simulink model "Final"  (R2021a)
settings: Solver=VariableStepAuto  StartTime=0.0  StopTime=1  RelTol=1e-3
undefined symbols (not defined in the file): Ion, Lithium
libraries: spsDiodeLib x7, spsSeriesRLCBranchLib x5, spsCurrentMeasurementLib x2, spsVoltageMeasurementLib x2, spsBatteryLib x1, spsMosfetLib x1, spsPVArrayLib x1, simulink x1, spsGroundLib x1, spsPermanentMagnetSynchronousMachineLib x1, spsThreePhaseVIMeasurementLib x1, spsWindTurbineLib x1
settings Model: Creator=Akashgowda  LastModifiedBy=Akashgowda

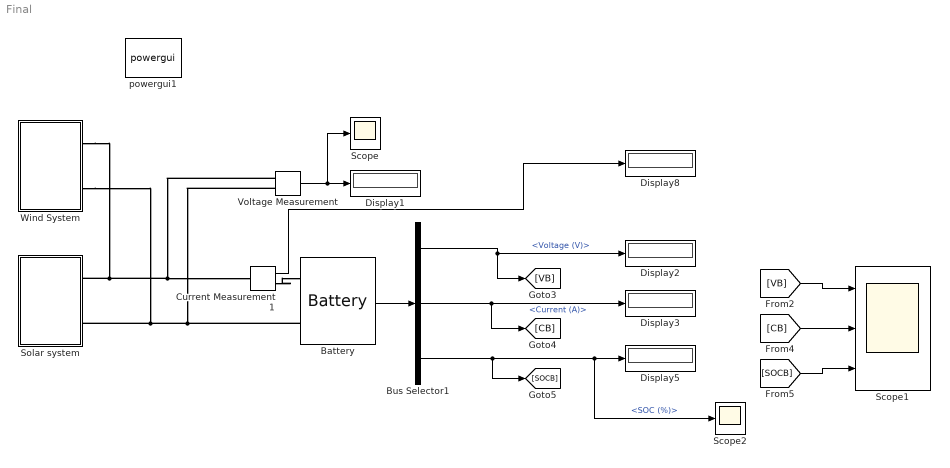
== system Final ==
  Battery : spsBatteryLib/Battery  BatType=Lithium-Ion  ShowTempParam=off  ThermalPreset=no  ShowAgeParam=off  NomV=12  NomQ=150  SOC=90  Batt_Tr=10  PresetModel=on  MaxQ=150  MinV=9  FullV=13.9678  Dis_rate=65.2174  R=0.0008  Normal_OP=135.6522  expZone="[12.9646      7.36957]"  current=[6.5 13 32.5]  Units=Time  Tci=20  NomT=20  T2=-30  MaxQ2=4.8  FullV2=7.1  Normal_OP2=5.655  expZone2="[6.58           1]"  Rca=0.6  ti=2000  Dp=0  Neq0=0  Tsim=1e6  Ta1=25  Qeol=5.4*0.9  Reol=0.013333*1.2  Char_age=[2.3478, 3]  Dis_age=[2.3478, 10]  N1=1500  N2=10500  N3=1000  N4=1400  Ta2=45  N5=950
  Bus Selector1 : BusSelector  OutputSignals=Voltage (V),Current (A),SOC (%)
  Current Measurement1 : spsCurrentMeasurementLib/Current Measurement  PhasorSimulation=off  OutputType=Complex  PSBequivalent=0
  Display{1..3,5,8} (5 alike) : Display
  Scope : Scope
  Scope1 : Scope  NumInputPorts=3
  Scope2 : Scope
  Solar system : Subsystem
  Voltage Measurement : spsVoltageMeasurementLib/Voltage Measurement  PhasorSimulation=off  OutputType=Complex  PSBequivalent=0
  Wind System : Subsystem
  powergui1 : spspowerguiLib/powergui  Priority=1  SimulationMode=Continuous  SampleTime=50e-6  frequency=60  Iterations=50  frequencyindice=0  Pbase=100e6  ErrMax=1e-4  UnitsV=kV  UnitsW=MW  buscounter=0  FunctionMessages=off  echomessages=off  EnableUseOfTLC=off  CurrentSourceSwitches=off  DisableSnubberDevices=off  DisableRonSwitches=off  DisableVfSwitches=off  DisplayEquations=off  AutomaticDiscreteSolvers=off  SolverType=Tustin/Backward Euler (TBE)  Interpol=off  ExternalGateDelay=off  methode=off  Ts=100  x0status=blocks  SPID=on  SwTol=0  HookPort=off  NonlinearTolerance=1e-4  nMaxIteration=100  ContinueOnMaxIteration=off  RestoreLinks=warning  ResistiveCurrentMeasurement=off  Frange=[0:2:500]  Ylog=off  Xlog=on  ShowGrid=off  save=off  variable=ZData  structure=0  ZoomFFT=off  StartTime=0.0  cycles=1  DisplayStyle=1  fundamental=60  FreqAxis=off  MaxFrequency=1000  frequencyindicesteady=1  RmsSteady=1  display=off
  wires:
  [VB] -> Scope1/1
  [SOCB] -> Scope1/3
  Bus Selector1/1 -> Display2/1, [VB]  "<Voltage (V)>"
  Bus Selector1/3 -> [SOCB], Scope2/1, Display5/1  "<SOC (%)>"
  Bus Selector1/2 -> [CB], Display3/1  "<Current (A)>"
  [CB] -> Scope1/2
  Battery/1 -> Bus Selector1/1
  Voltage Measurement/1 -> Scope/1, Display1/1
  Current Measurement1/1 -> Display8/1
  connections:
  Wind System/RConn2 -- Battery/LConn2 -- Voltage Measurement/LConn2 -- Solar system/RConn2
  Wind System/RConn1 -- Current Measurement1/LConn1 -- Voltage Measurement/LConn1 -- Solar system/RConn1
  Current Measurement1/RConn1 -- Battery/LConn1

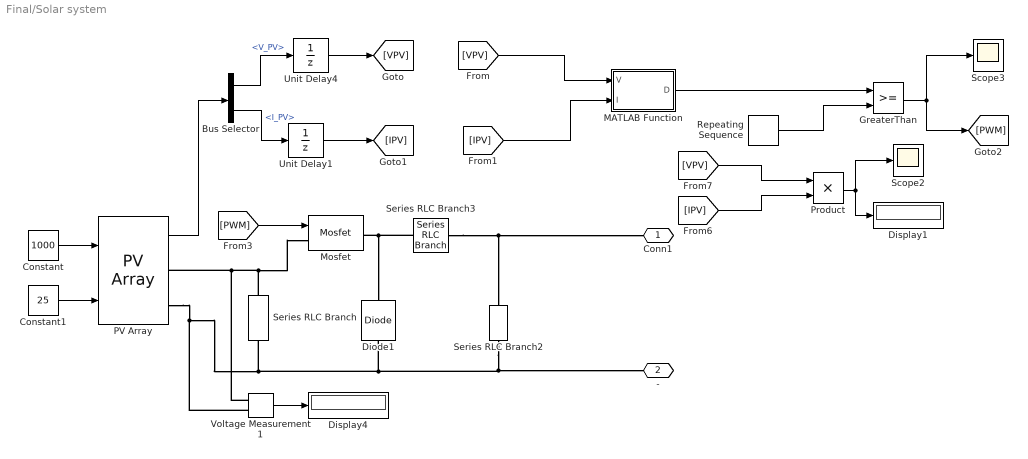
== system Final/Solar system ==
  Bus Selector : BusSelector  OutputSignals=V_PV,I_PV
  Constant : Constant  Value=1000
  Constant1 : Constant  Value=25
  Diode1 : spsDiodeLib/Diode  Ron=0.001  Lon=0  Vf=0.8  IC=0  UseSnubber=0  Rs=500  Cs=250e-9  Measurements=off
  Display1 : Display
  Display4 : Display
  GreaterThan : RelationalOperator  OutDataTypeStr=boolean  RndMeth=Simplest
  MATLAB Function : MATLAB Function  TreatAsAtomicUnit=on
  Mosfet : spsMosfetLib/Mosfet  Ron=0.1  Lon=0  Rd=0.01  Vfd=0  IC=0  Rs=1e5  Cs=inf  Measurements=off
  PV Array : spsPVArrayLib/PV Array  Npar=1  Nser=1  PlotType=array @ 25 deg.C & specified irradiances  S_vec="[ 1000  500  100 ]"  Temp_C_vec="[ 45 25  ]"  ModuleName=User-defined  PlotWhenSelected=off  Pm=213.15  Ncell=60  Voc=36.3  Isc=7.84  Vm=29  Im=7.35  beta_Voc_pc=-0.36099  alpha_Isc_pc=0.102  beta_Voc=-0.13104  alpha_Isc=0.0079968  IL=7.8654  I0=2.9273e-10  nI=0.98119  Rsh=313.0553  Rs=0.39381  RobustModel=off  RobustCellTemperature=313.3991  BAL=on  Tc=1e-6  Tfilter=5e-5
  Product : Product
  Repeating Sequence : simulink/Sources/Repeating Sequence  rep_seq_t=[0 0.0002]  rep_seq_y=[0 1]
  Scope2 : Scope
  Scope3 : Scope
  Series RLC Branch : spsSeriesRLCBranchLib/Series RLC Branch  LConnTagsString=__new0  RConnTagsString=__new0  BranchType=RC  Resistance=0.0001  Inductance=1e-3  SetiL0=off  InitialCurrent=0  Capacitance=1000e-6  Setx0=off  InitialVoltage=0  Measurements=None
  Series RLC Branch2 : spsSeriesRLCBranchLib/Series RLC Branch  LConnTagsString=__new0  RConnTagsString=__new0  BranchType=C  Resistance=1  Inductance=1e-3  SetiL0=off  InitialCurrent=0  Capacitance=369.79e-6  Setx0=off  InitialVoltage=0  Measurements=None
  Series RLC Branch3 : spsSeriesRLCBranchLib/Series RLC Branch  LConnTagsString=__new0  RConnTagsString=__new0  BranchType=L  Resistance=1  Inductance=772.64e-6  SetiL0=off  InitialCurrent=0  Capacitance=1e-6  Setx0=off  InitialVoltage=0  Measurements=None
  Unit Delay1 : UnitDelay  SampleTime=1e-4  HasFrameUpgradeWarning=on
  Unit Delay4 : UnitDelay  SampleTime=1e-4  HasFrameUpgradeWarning=on
  Voltage Measurement1 : spsVoltageMeasurementLib/Voltage Measurement  PhasorSimulation=off  OutputType=Complex  PSBequivalent=0
  Conn1 : PMIOPort  Side=Right
  - : PMIOPort  Port=2  Side=Right
  wires:
  Voltage Measurement1/1 -> Display4/1
  Constant/1 -> PV Array/1
  Bus Selector/2 -> Unit Delay1/1  "<I_PV>"
  Product/1 -> Display1/1, Scope2/1
  [IPV] -> Product/2
  PV Array/1 -> Bus Selector/1
  Constant1/1 -> PV Array/2
  Unit Delay4/1 -> [VPV]
  [VPV] -> Product/1
  Bus Selector/1 -> Unit Delay4/1  "<V_PV>"
  [VPV] -> MATLAB Function/1(V)
  Unit Delay1/1 -> [IPV]
  MATLAB Function/1(D) -> GreaterThan/1
  [IPV] -> MATLAB Function/2(I)
  Repeating Sequence/1 -> GreaterThan/2
  [PWM] -> Mosfet/1
  GreaterThan/1 -> Scope3/1, [PWM]
  connections:
  Series RLC Branch2/RConn1 -- PV Array/RConn2 -- Voltage Measurement1/LConn2 -- Series RLC Branch/RConn1 -- Diode1/LConn1 -- -/RConn1
  PV Array/RConn1 -- Series RLC Branch/LConn1 -- Mosfet/LConn1 -- Voltage Measurement1/LConn1
  Series RLC Branch3/RConn1 -- Mosfet/RConn1 -- Diode1/RConn1
  Series RLC Branch3/LConn1 -- Conn1/RConn1 -- Series RLC Branch2/LConn1

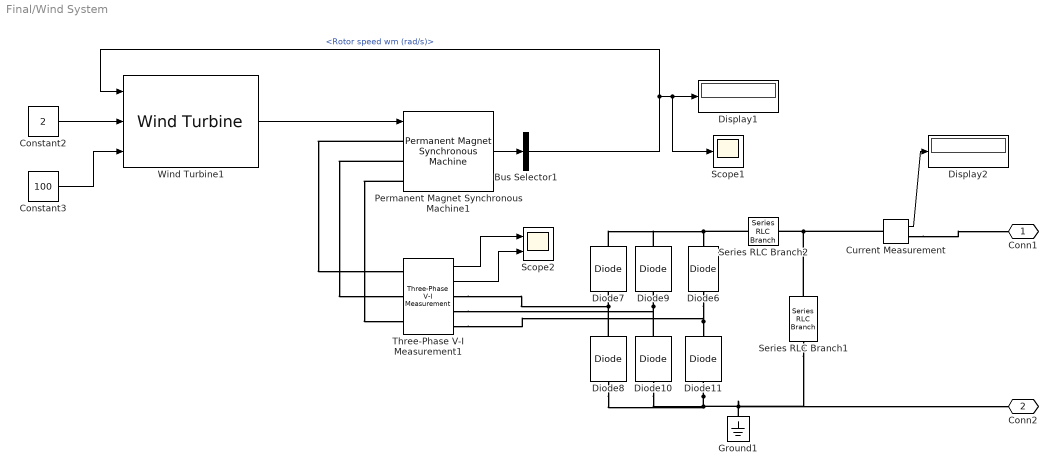
== system Final/Wind System ==
  Bus Selector1 : BusSelector  OutputSignals=Rotor speed wm (rad/s)
  Constant2 : Constant  Value=2
  Constant3 : Constant  Value=100
  Current Measurement : spsCurrentMeasurementLib/Current Measurement  PhasorSimulation=off  OutputType=Complex  PSBequivalent=0
  Diode{6..11} (6 alike) : spsDiodeLib/Diode  Ron=0.001  Lon=0  Vf=0.8  IC=0  UseSnubber=0  Rs=500  Cs=250e-9  Measurements=off
  Display1 : Display
  Display2 : Display
  Ground1 : spsGroundLib/Ground  LConnTagsString=a
  Permanent Magnet Synchronous Machine1 : spsPermanentMagnetSynchronousMachineLib/Permanent Magnet Synchronous Machine  NbPhases=3  FluxDistribution=Sinusoidal  RotorType=Round  MechanicalLoad=Torque Tm  PresetModel=No  ShowDetailedParameters=on  MeasurementBus=off  Resistance=0.0485  Inductance=8.5e-3  dqInductances=[8.5e-3,8.5e-3]  La=0.000395  MachineConstant=Flux linkage established by magnets (V.s)  Flux=0.1194  VoltageCst=86.6271  TorqueCst=0.7164  Flat=120  Mechanical=[0.0027 0.0004924 4 0]  PolePairs=4  InitialConditions=[0,0, 0,0]  InitialConditions5ph=[0 0 0 0 0 0]  RefAngle=90 degrees behind phase A axis (modified Park)  IterativeDiscreteModel=Trapezoidal non iterative  TsBlock=-1  TsPowergui=0
  Scope1 : Scope
  Scope2 : Scope  NumInputPorts=2
  Series RLC Branch1 : spsSeriesRLCBranchLib/Series RLC Branch  LConnTagsString=__new0  RConnTagsString=__new0  BranchType=C  Resistance=1  Inductance=1e-3  SetiL0=off  InitialCurrent=0  Capacitance=200e-6  Setx0=off  InitialVoltage=0  Measurements=None
  Series RLC Branch2 : spsSeriesRLCBranchLib/Series RLC Branch  LConnTagsString=__new0  RConnTagsString=__new0  BranchType=L  Resistance=1  Inductance=1e-3  SetiL0=off  InitialCurrent=0  Capacitance=200e-6  Setx0=off  InitialVoltage=0  Measurements=None
  Three-Phase V-I Measurement1 : spsThreePhaseVIMeasurementLib/Three-Phase V-I Measurement  VoltageMeasurement=phase-to-ground  SetLabelV=off  LabelV=Vabc  Vpu=off  VpuLL=off  CurrentMeasurement=yes  SetLabelI=off  LabelI=Iabc  Ipu=off  Pbase=100e6  Vbase=500e3  OutputType=Complex  PhasorSimulation=off  PSBequivalent=0
  Wind Turbine1 : spsWindTurbineLib/Wind Turbine  Pnom=1.5e6  Pelec_base=1.5e6/0.9  wind_base=12  P_wind_base=0.73  speed_nom=1.2  pitch_angle=0  c1_c6="[0.51763          116          0.4            5           21     0.006795]"  cp_nom=0.48  lambda_nom=8.1
      settings: SourceProductBaseCode=PS
  Conn1 : PMIOPort  Side=Right
  Conn2 : PMIOPort  Port=2  Side=Right
  wires:
  Constant2/1 -> Wind Turbine1/2
  Bus Selector1/1 -> Wind Turbine1/1, Scope1/1, Display1/1  "<Rotor speed wm (rad/s)>"
  Three-Phase V-I Measurement1/2 -> Scope2/2
  Wind Turbine1/1 -> Permanent Magnet Synchronous Machine1/1
  Constant3/1 -> Wind Turbine1/3
  Three-Phase V-I Measurement1/1 -> Scope2/1
  Permanent Magnet Synchronous Machine1/1 -> Bus Selector1/1
  Current Measurement/1 -> Display2/1
  connections:
  Diode6/RConn1 -- Series RLC Branch2/LConn1 -- Diode7/RConn1 -- Diode9/RConn1
  Diode7/LConn1 -- Diode8/RConn1 -- Three-Phase V-I Measurement1/RConn1
  Diode9/LConn1 -- Three-Phase V-I Measurement1/RConn2 -- Diode10/RConn1
  Diode11/LConn1 -- Series RLC Branch1/RConn1 -- Conn2/RConn1 -- Ground1/LConn1 -- Diode8/LConn1 -- Diode10/LConn1
  Series RLC Branch1/LConn1 -- Current Measurement/LConn1 -- Series RLC Branch2/RConn1
  Diode11/RConn1 -- Diode6/LConn1 -- Three-Phase V-I Measurement1/RConn3
  Permanent Magnet Synchronous Machine1/LConn1 -- Three-Phase V-I Measurement1/LConn1
  Permanent Magnet Synchronous Machine1/LConn2 -- Three-Phase V-I Measurement1/LConn2
  Permanent Magnet Synchronous Machine1/LConn3 -- Three-Phase V-I Measurement1/LConn3
  Current Measurement/RConn1 -- Conn1/RConn1

== matlab function Final/Solar system/MATLAB Function ==
  data: V input; D output; I input
function D = Duty_cycle(V, I)

Dmax = 0.95;
Dmin = 0;
Dinit = 0.95;
deltaD = 0.0001;

persistent Vold Pold Dold;
dataType = 'double';

if isempty(Vold)
    Vold =0;
    Pold=0;
    Dold=Dinit;
end

P = V*I;
dV = V-Vold;
dP = P-Pold;

if dP ~= 0
    if dP<0
        if dV<0
            D = Dold - deltaD;
        else
            D = Dold - deltaD;
        end
    else
        if dV<0
            D = Dold + deltaD;
        else
            D = Dold - deltaD;
        end
    end
else D = Dold
end
if D >= Dmax || D < Dmin
    D = Dold
end
Dold = D;
Vold=V;
Pold=P;
